simulink model "openMHA_test_FFT_to_gain"  (R2020b)
settings: Solver=VariableStepAuto  StartTime=0.0  StopTime=stop_time  RelTol=1e-3
InitFcn:
  | test_FFT_to_gain_init
StopFcn:
  | test_FFT_to_gain_stop
values from neighbouring files (symbols this model uses):
  band_edges = [band_edges mirrored_band_edges]    [test_FFT_to_gain_init.m]    (also in test_db_lookup_gain_fpga_init.m = calculate_band_edges(ef, num_bins, binwidth, num_bands); test_db_lookup_init.m = calculate_band_edges(ef, num_bins, binwidth, num_bands); test_gaintable_init.m = calculate_band_edges(ef, num_bins, binwidth, num_bands); test_init.m = calculate_band_edges(ef, num_bins, binwidth, num_bands))
  buf_a = 65.*ones(num_bands,1)    [test_FFT_to_gain_init.m]    (also in test_ar_filter_dualport_init.m; test_db_ar_gaintable_init.m)
  delay_memory_size = 2^system_delay_memory    [test_FFT_to_gain_init.m]    (also in test_state_gainapp_cbuf_init.m)
  FFTsize = 256    [test_FFT_to_gain_init.m]    (also in test_ar_filter_gaintable_init.m; test_db_ar_gaintable_init.m; test_db_lookup_gain_fpga_init.m; test_db_lookup_init.m)
  gainapp_dp_memory = log2(num_bands) + 1    [test_FFT_to_gain_init.m]    (also in test_state_gainapp_cbuf_init.m)
  num_bands = 8    [calculate_gaintable.m]    (also in test_FFT_to_gain_init.m = 2; test_ar_filter_dualport_init.m = 2; test_db_ar_gaintable_init.m = 2; test_db_lookup_gain_fpga_init.m = 9)
  num_bins = FFTsize/2 + 1    (= 129)    [test_FFT_to_gain_init.m]    (also in test_ar_filter_gaintable_init.m; test_db_ar_gaintable_init.m; test_db_lookup_gain_fpga_init.m; test_db_lookup_init.m)
  system_delay = 6 + max(band_sizes)    [test_FFT_to_gain_init.m]    (also in test_state_gainapp_cbuf_init.m = max(band_sizes))
  table_length = length(gtdata)    [calculate_gaintable.m]    (also in test_FFT_to_gain_init.m; test_ar_filter_gaintable_init.m; test_db_ar_gaintable_init.m; test_db_lookup_gain_fpga_init.m)
  X_high = 93    [test_FFT_to_gain_init.m]    (also in test_ar_filter_gaintable_init.m = 95; test_db_ar_gaintable_init.m; test_db_lookup_gain_fpga_init.m = 95; test_db_lookup_init.m = 95)
  xIn = [4.65661287308e-10 5.23868948221e-10 5.82076609135e-10 6.40284270048e-10 6.98491930962e-10 7.56699591875e-10 8.14907252789e-10 8.73114913702e-10 9.31322574615e-10 1.04773789644e-09 1.16415321827e-09 1.2805685401e-09 ... (256 elements, 1x256)]    [openMHA_test_db_lookup_gain_Programmable Look-Up Table_init.mat]    (also in openMHA_test_db_lookup_gain_Programmable Lookup Table dB_init.mat = [4.65661287308e-10 4.72937244922e-10 4.80213202536e-10 4.874)
libraries: dspsrcs4 x9, hdlsllib x8, simulink x4, FPGA_Open_Speech_Tools x3
(part 2 of 2)

== matlab function openMHA_test_FFT_to_gain/Fequency Band Compression/Intensity/Frequency Band Intensity Accumulator ==
  data: bin_intensity input; level_in output fixdt(1,Wbits,Fbits); accumulator_reset input; bin_num input; num_bins input
function level_in = accumulate_band(bin_intensity, accumulator_reset, bin_num, num_bins)

% Accumulates the bin intensities until a new frequency band is detected.
% Takes in the current frequency bin intensity, an accumulator reset
% control signal, bin number and number of frequency bins. If the 
% accumulator_reset is true, the sum is reset starting with the current 
% frequency bin intensity. Unless a DC or Nyquist bin is detected, a
% logical shift left is executed to apply a gain of two to the current
% bin_intensity, which accounts for negative frequencies.

persistent total;

if isempty(total)
    total = fi(0,1,40,32);
end

if bin_num == 0 || bin_num == num_bins-1
    dc_nyquist = true;
else
    dc_nyquist = false;
end

if accumulator_reset == true && dc_nyquist == true
    total = fi(bin_intensity,1,40,32);
    level_in = total;
elseif accumulator_reset == true && dc_nyquist == false
    total = bitsll(fi(bin_intensity,1,40,32),fi(1));
    level_in = total;
elseif accumulator_reset == false && dc_nyquist == true
    total = fi(total + fi(bin_intensity,1,40,32),1,40,32);
    level_in = total;
elseif accumulator_reset == false && dc_nyquist == false
    total = fi(total + bitsll(fi(bin_intensity,1,40,32),fi(1)),1,40,32);
    level_in = total;
else
    total = fi(0,1,40,32);
    error('Incorrect Logic in accumulate_band function!');
end
